simulink model "swingup20112025moi2018a"  (R2018a)
settings: Solver=VariableStepAuto  StartTime=0.0  StopTime=20  RelTol=1e-3
values from neighbouring files (symbols this model uses):
  alphaldotini = 0    [thamsosswingup20112025.m]
  alphalini = 0*pi/180    (= 0)    [thamsosswingup20112025.m]
  bp = 0.005    [calculate_new_K.m]    (also in thamsosswingup20112025.m; verify_quanser_equations.m)
  br = 0.0015    [calculate_new_K.m]    (also in thamsosswingup20112025.m; verify_quanser_equations.m)
  g = 9.81    [calculate_new_K.m]    (also in swingup_control.m = params.g; thamsosswingup20112025.m; verify_quanser_equations.m)
  Jp = mp*(Lp^2)/3    (= 0.000133128)    [calculate_new_K.m]    (also in thamsosswingup20112025.m; verify_quanser_equations.m)
  Jp_cm = params.Jp_cm    [swingup_control.m]    (also in thamsosswingup20112025.m = 3.3282e-05)
  Jr = (mr*r^2)/3    (= 0.000228791666667)    [calculate_new_K.m]    (also in thamsosswingup20112025.m; verify_quanser_equations.m)
  K = (R \ B') * S    [calculate_new_K.m]    (also in lqr_custom.m = R \ (B' * S); swingup_control.m = params.K; thamsosswingup20112025.m = [-3.1623   84.6410   -3.1854    9.2746])
  km = 0.042    [calculate_new_K.m]    (also in thamsosswingup20112025.m)
  Kt = 0.042    [calculate_new_K.m]    (also in thamsosswingup20112025.m)
  l = Lp/2    (= 0.0645)    [calculate_new_K.m]    (also in swingup_control.m = params.l; thamsosswingup20112025.m; verify_quanser_equations.m)
  mp = 0.024    [calculate_new_K.m]    (also in swingup_control.m = params.mp; thamsosswingup20112025.m; verify_quanser_equations.m)
  mr = 0.095    [calculate_new_K.m]    (also in thamsosswingup20112025.m; verify_quanser_equations.m)
  r = 0.085    [calculate_new_K.m]    (also in thamsosswingup20112025.m; verify_quanser_equations.m)
  Rm = 8.4    [calculate_new_K.m]    (also in thamsosswingup20112025.m)
  theta_max = 180*pi/180    (= 3.14159265359)    [thamsosswingup20112025.m]
  thetadotini = 0    [thamsosswingup20112025.m]
  thetaini = 0*pi/180    (= 0)    [thamsosswingup20112025.m]
undefined symbols (not defined in the file or in its folder): Km
libraries: simulink x4, simulink_extras x3
settings Model: Creator=ASUS  LastModifiedBy=ASUS
settings SolverCC: ZeroCrossAlgorithm=Adaptive
settings DataIOCC: ReturnWorkspaceOutputs=on
settings DebuggingCC: IgnoredZcDiagnostic=none  UnconnectedInputMsg=none  UnconnectedOutputMsg=none  UnconnectedLineMsg=none
settings ModelReferenceCC: EnableRefExpFcnMdlSchedulingChecks=off
settings SFSimCC: SimUseLocalCustomCode=on
settings RTWCC: Description=Generic Real-Time Target  RTWUseLocalCustomCode=on

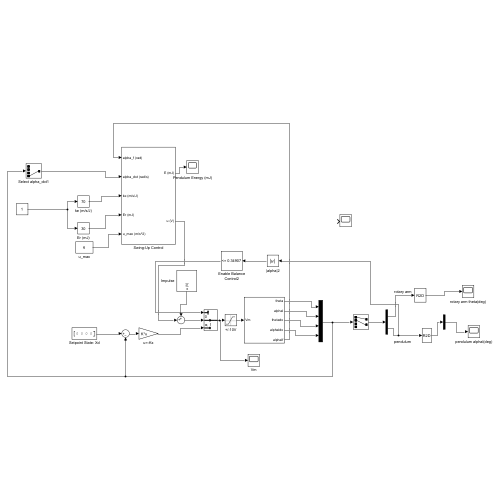
[thumbnail: Simulink's stored preview of the top-level diagram]
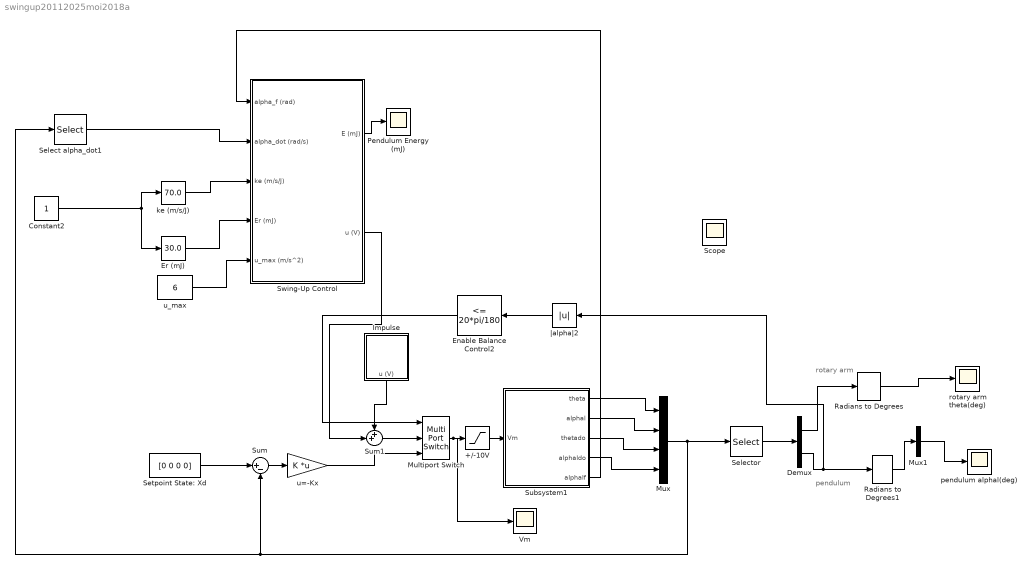
== system swingup20112025moi2018a ==
  note: pendulum
  note: rotary arm
  +/-10V : Saturate  UpperLimit=15  LowerLimit=-15
  Constant2 : Constant
  Demux : Demux  Outputs=2
  Enable Balance Control2 : simulink/Logic and Bit Operations/Compare To Constant  relop=<=  const=20*pi/180  OutDataTypeStr=uint8  ZeroCross=off
  Er (mJ) : simulink/Math Operations/Slider Gain  gain=30.0  low=0  high=100
  Impulse : Subsystem
  Multiport Switch : MultiPortSwitch  DataPortOrder=Zero-based contiguous  Inputs=2  zeroidx=on
  Mux : Mux
  Mux1 : Mux  Inputs=1
  Pendulum Energy (mJ) : Scope
  Radians to Degrees : simulink_extras/Transformations/Radians to Degrees
  Radians to Degrees1 : simulink_extras/Transformations/Radians to Degrees
  Scope : Scope
  Select alpha_dot1 : Selector  InputPortWidth=4  IndexOptions=Index vector (dialog)  Indices=[4]  OutputSizes=1
  Selector : Selector  InputPortWidth=4  IndexOptions=Index vector (dialog)  Indices=[1 2]  OutputSizes=1
  Setpoint State: Xd : Constant  Value=[0 0 0 0]
  Subsystem1 : Subsystem
  Sum : Sum  Inputs=|+-
  Sum1 : Sum  Inputs=++|
  Swing-Up Control : Subsystem
  Vm : Scope
  ke (m/s/J) : simulink/Math Operations/Slider Gain  gain=70.0  low=0  high=100
  pendulum alphal(deg) : Scope
  rotary arm theta(deg) : Scope
  u=-Kx : Gain  Gain=K  Multiplication=Matrix(K*u)
  u_max : Constant  Value=6
  |alpha|2 : Abs
  wires:
  Radians to Degrees1/1 -> Mux1/1
  Demux/1 -> Radians to Degrees/1
  u=-Kx/1 -> Multiport Switch/3
  Selector/1 -> Demux/1
  Enable Balance Control2/1 -> Multiport Switch/1
  Radians to Degrees/1 -> rotary arm theta(deg)/1
  Sum1/1 -> Multiport Switch/2
  Mux1/1 -> pendulum alphal(deg)/1
  Demux/2 -> |alpha|2/1, Radians to Degrees1/1
  Multiport Switch/1 -> Vm/1, +/-10V/1
  Subsystem1/3(thetado) -> Mux/3
  Subsystem1/2(alphal) -> Mux/2
  Subsystem1/1(theta) -> Mux/1
  |alpha|2/1 -> Enable Balance Control2/1
  Mux/1 -> Selector/1, Select alpha_dot1/1, Sum/2
  Subsystem1/4(alphaldo) -> Mux/4
  Swing-Up Control/1(E (mJ)) -> Pendulum Energy (mJ)/1
  Impulse/1(u (V)) -> Sum1/1
  Er (mJ)/1 -> Swing-Up Control/4(Er (mJ))
  ke (m/s/J)/1 -> Swing-Up Control/3(ke (m/s/J))
  Constant2/1 -> Er (mJ)/1, ke (m/s/J)/1
  u_max/1 -> Swing-Up Control/5(u_max (m/s^2))
  Setpoint State: Xd/1 -> Sum/1
  Sum/1 -> u=-Kx/1
  Select alpha_dot1/1 -> Swing-Up Control/2(alpha_dot (rad/s))
  Swing-Up Control/2(u (V)) -> Sum1/2
  +/-10V/1 -> Subsystem1/1(Vm)
  Subsystem1/5(alphalf) -> Swing-Up Control/1(alpha_f (rad))

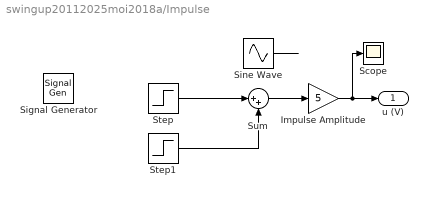
== system swingup20112025moi2018a/Impulse ==
  Impulse Amplitude : Gain  Gain=5
  Scope : Scope
  Signal Generator : SignalGenerator  WaveForm=square  Amplitude=5  Frequency=0.125
  Sine Wave : Sin  Amplitude=6  SampleTime=0
  Step : Step  SampleTime=0
  Step1 : Step  Time=1.1  After=-1  SampleTime=0
  Sum : Sum  Inputs=|++
  u (V) : Outport  VectorParamsAs1DForOutWhenUnconnected=off
  wires:
  Step1/1 -> Sum/2
  Step/1 -> Sum/1
  Sine Wave/1 -> ?
  Impulse Amplitude/1 -> Scope/1, u (V)/1
  Sum/1 -> Impulse Amplitude/1

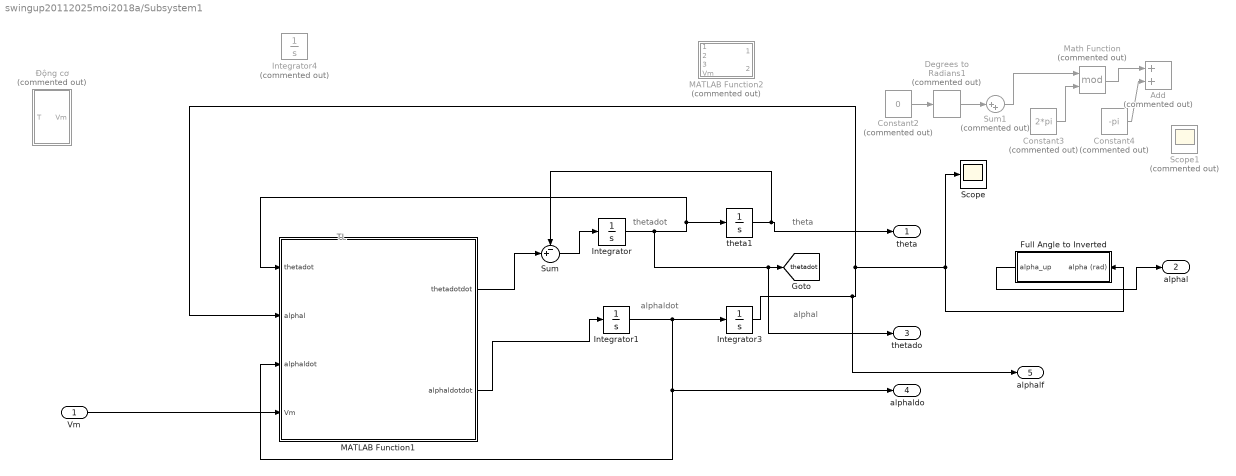
== system swingup20112025moi2018a/Subsystem1 ==
  note: theta
  note: alphaldot
  note: TL
  note: thetadot
  note: alphal
  Vm : Inport
  Add : Sum  Commented=on
  Constant2 : Constant  Commented=on  Value=0
  Constant3 : Constant  Commented=on  Value=2*pi
  Constant4 : Constant  Commented=on  Value=-pi
  Degrees to Radians1 : simulink_extras/Transformations/Degrees to Radians  Commented=on
  Full Angle to Inverted : Subsystem
  Integrator : Integrator  InitialCondition=thetadotini
  Integrator1 : Integrator  InitialCondition=alphaldotini
  Integrator3 : Integrator  InitialCondition=alphalini
  Integrator4 : Integrator  Commented=on  InitialCondition=thetaini
  MATLAB Function1 : MATLAB Function  TreatAsAtomicUnit=on
  MATLAB Function2 : MATLAB Function  Commented=on  TreatAsAtomicUnit=on
  Math Function : Math  Commented=on  Operator=mod  SaturateOnIntegerOverflow=on
  Scope : Scope
  Scope1 : Scope  Commented=on
  Sum : Sum  Inputs=-+|
  Sum1 : Sum  Commented=on  Inputs=|++
  theta1 : Integrator  LimitOutput=on  UpperSaturationLimit=theta_max  LowerSaturationLimit=-theta_max
  Động cơ : Subsystem  Commented=on
  theta : Outport
  alphal : Outport  Port=2
  thetado : Outport  Port=3
  alphaldo : Outport  Port=4
  alphalf : Outport  Port=5
  tag scope: thetadot=global
  wires:
  Integrator/1 -> thetado/1, [thetadot], MATLAB Function1/1(thetadot), theta1/1
  theta1/1 -> Sum/1, theta/1
  Integrator1/1 -> MATLAB Function1/3(alphaldot), alphaldo/1, Integrator3/1
  MATLAB Function1/1(thetadotdot) -> Sum/2
  Constant3/1 -> Math Function/2
  Constant4/1 -> Add/2
  Constant2/1 -> Degrees to Radians1/1
  Math Function/1 -> Add/1
  Sum1/1 -> Math Function/1
  Degrees to Radians1/1 -> Sum1/1
  Sum/1 -> Integrator/1
  Vm/1 -> MATLAB Function1/4(Vm)
  Integrator3/1 -> alphalf/1, Scope/1, Full Angle to Inverted/1(alpha (rad)), MATLAB Function1/2(alphal)
  MATLAB Function1/2(alphaldotdot) -> Integrator1/1
  Full Angle to Inverted/1(alpha_up) -> alphal/1

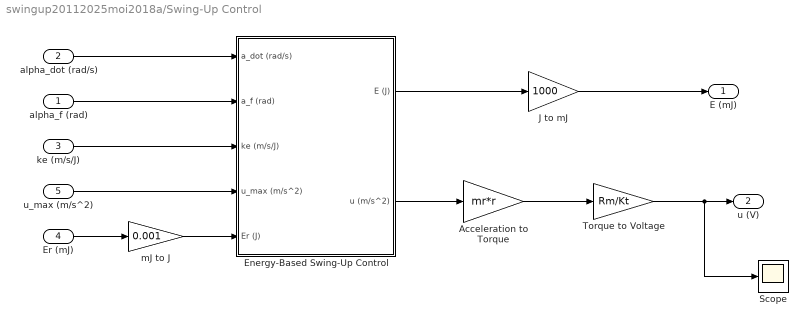
== system swingup20112025moi2018a/Swing-Up Control ==
  alpha_f (rad) : Inport
  alpha_dot (rad/s) : Inport  Port=2
  ke (m/s/J) : Inport  Port=3
  Er (mJ) : Inport  Port=4
  u_max (m/s^2) : Inport  Port=5
  Acceleration to Torque : Gain  Gain=mr*r
  Energy-Based Swing-Up Control : Subsystem
  J to mJ : Gain  Gain=1000
  Scope : Scope
  Torque to Voltage : Gain  Gain=Rm/Kt
  mJ to J : Gain  Gain=0.001
  E (mJ) : Outport  VectorParamsAs1DForOutWhenUnconnected=off
  u (V) : Outport  Port=2  VectorParamsAs1DForOutWhenUnconnected=off
  wires:
  Energy-Based Swing-Up Control/2(u (m/s^2)) -> Acceleration to Torque/1
  Energy-Based Swing-Up Control/1(E (J)) -> J to mJ/1
  alpha_f (rad)/1 -> Energy-Based Swing-Up Control/2(a_f (rad))
  ke (m/s/J)/1 -> Energy-Based Swing-Up Control/3(ke (m/s/J))
  u_max (m/s^2)/1 -> Energy-Based Swing-Up Control/4(u_max (m/s^2))
  Acceleration to Torque/1 -> Torque to Voltage/1
  Er (mJ)/1 -> mJ to J/1
  J to mJ/1 -> E (mJ)/1
  Torque to Voltage/1 -> Scope/1, u (V)/1
  alpha_dot (rad/s)/1 -> Energy-Based Swing-Up Control/1(a_dot (rad/s))
  mJ to J/1 -> Energy-Based Swing-Up Control/5(Er (J))

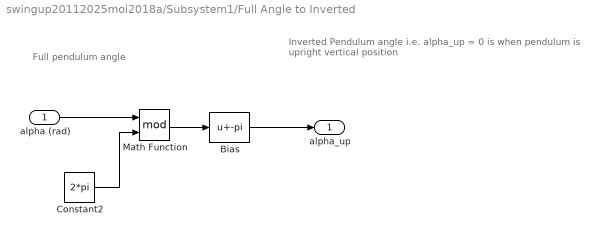
== system swingup20112025moi2018a/Subsystem1/Full Angle to Inverted ==
  note: Inverted Pendulum angle
      | i.e. alpha_up = 0 is when pendulum is upright vertical position
  note: Full pendulum angle
  alpha (rad) : Inport
  Bias : Bias  Bias=-pi
  Constant2 : Constant  Value=2*pi
  Math Function : Math  Operator=mod  SaturateOnIntegerOverflow=on
  alpha_up : Outport  VectorParamsAs1DForOutWhenUnconnected=off
  wires:
  Constant2/1 -> Math Function/2
  alpha (rad)/1 -> Math Function/1
  Bias/1 -> alpha_up/1
  Math Function/1 -> Bias/1

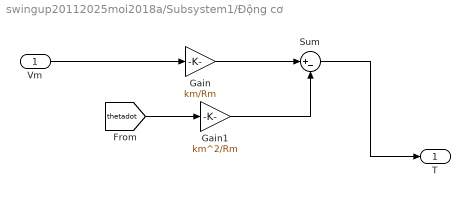
== system swingup20112025moi2018a/Subsystem1/Động cơ ==
  Vm : Inport
  Gain : Gain  Gain=km/Rm
  Gain1 : Gain  Gain=km^2/Rm
  Sum : Sum  Inputs=|+-
  T : Outport
  wires:
  Sum/1 -> T/1
  Gain1/1 -> Sum/2
  Gain/1 -> Sum/1
  Vm/1 -> Gain/1
  [thetadot] -> Gain1/1

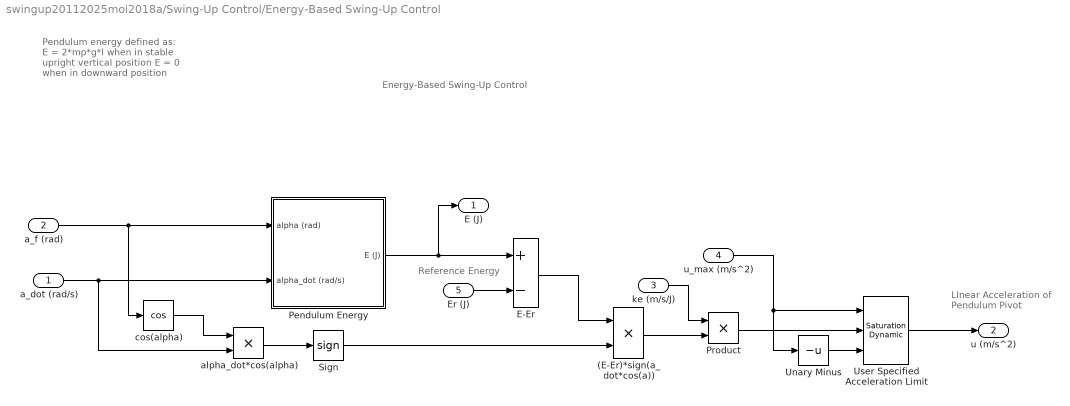
== system swingup20112025moi2018a/Swing-Up Control/Energy-Based Swing-Up Control ==
  note: Energy-Based Swing-Up Control
  note: LInear Acceleration of
      | Pendulum Pivot
  note: Reference Energy
  note: Pendulum energy defined as:
      | E = 2*mp*g*l when in stable upright vertical position
      | E = 0 when in downward position
  a_dot (rad/s) : Inport
  a_f (rad) : Inport  Port=2
  ke (m/s/J) : Inport  Port=3
  u_max (m/s^2) : Inport  Port=4
  Er (J) : Inport  Port=5
  (E-Er)*sign(a_dot*cos(a)) : Product  RndMeth=Zero
  E-Er : Sum  Inputs=+-
  Pendulum Energy : Subsystem
  Product : Product  RndMeth=Zero
  Sign : Signum
  Unary Minus : UnaryMinus
  User Specified Acceleration Limit : simulink/Discontinuities/Saturation Dynamic  OutMin=[]  OutMax=[]  OutDataTypeStr=Inherit: Same as second input  OutDataType=fixdt(1, 16)  OutScaling=2^-10  DoSatur=off
  alpha_dot*cos(alpha) : Product  RndMeth=Zero
  cos(alpha) : Trigonometry  Operator=cos
  E (J) : Outport  VectorParamsAs1DForOutWhenUnconnected=off
  u (m/s^2) : Outport  Port=2  VectorParamsAs1DForOutWhenUnconnected=off
  wires:
  a_f (rad)/1 -> Pendulum Energy/1(alpha (rad)), cos(alpha)/1
  Sign/1 -> (E-Er)*sign(a_dot*cos(a))/2
  alpha_dot*cos(alpha)/1 -> Sign/1
  cos(alpha)/1 -> alpha_dot*cos(alpha)/1
  E-Er/1 -> (E-Er)*sign(a_dot*cos(a))/1
  Pendulum Energy/1(E (J)) -> E (J)/1, E-Er/1
  a_dot (rad/s)/1 -> alpha_dot*cos(alpha)/2, Pendulum Energy/2(alpha_dot (rad/s))
  (E-Er)*sign(a_dot*cos(a))/1 -> Product/2
  Er (J)/1 -> E-Er/2
  ke (m/s/J)/1 -> Product/1
  Product/1 -> User Specified Acceleration Limit/2
  u_max (m/s^2)/1 -> User Specified Acceleration Limit/1, Unary Minus/1
  Unary Minus/1 -> User Specified Acceleration Limit/3
  User Specified Acceleration Limit/1 -> u (m/s^2)/1

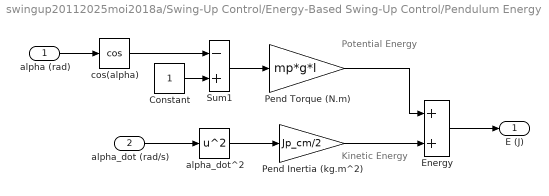
== system swingup20112025moi2018a/Swing-Up Control/Energy-Based Swing-Up Control/Pendulum Energy ==
  note: Kinetic Energy
  note: Potential Energy
  alpha (rad) : Inport
  alpha_dot (rad/s) : Inport  Port=2
  Constant : Constant
  Energy : Sum  SaturateOnIntegerOverflow=on
  Pend Inertia (kg.m^2) : Gain  Gain=Jp_cm/2
  Pend Torque (N.m) : Gain  Gain=mp*g*l
  Sum1 : Sum  Inputs=-+  SaturateOnIntegerOverflow=on
  alpha_dot^2 : Math  Operator=square  SaturateOnIntegerOverflow=on
  cos(alpha) : Trigonometry  Operator=cos
  E (J) : Outport  VectorParamsAs1DForOutWhenUnconnected=off
  wires:
  Sum1/1 -> Pend Torque (N.m)/1
  Constant/1 -> Sum1/2
  Pend Inertia (kg.m^2)/1 -> Energy/2
  alpha_dot^2/1 -> Pend Inertia (kg.m^2)/1
  Pend Torque (N.m)/1 -> Energy/1
  alpha (rad)/1 -> cos(alpha)/1
  alpha_dot (rad/s)/1 -> alpha_dot^2/1
  Energy/1 -> E (J)/1
  cos(alpha)/1 -> Sum1/1

== matlab function swingup20112025moi2018a/Subsystem1/MATLAB Function1 ==
  data: thetadotdot output; alphaldotdot output; thetadot input; alphal input; alphaldot input; Vm input; Jr parameter; br parameter; bp parameter; g parameter; l parameter; mp parameter; r parameter; Jp parameter; Kt parameter; Rm parameter; km parameter
function [thetadotdot,alphaldotdot] = fcn(thetadot,alphal, alphaldot,Vm,Jr, br, bp, g, l, mp, r, Jp,Kt, Rm, km)
 
thetadotdot = (Jp*(Kt/Rm)*(Vm-km*thetadot) - Jp*br*thetadot - 2*Jp^2*alphaldot*thetadot*cos(alphal)*sin(alphal) + alphaldot*bp*l*mp*r*cos(alphal) + g*l^2*mp^2*r*cos(alphal)*sin(alphal) + Jp*alphaldot^2*l*mp*r*sin(alphal) - Jp*l*mp*r*thetadot^2*cos(alphal)^2*sin(alphal))/(Jp^2*sin(alphal)^2 + Jr*Jp - l^2*mp^2*r^2*cos(alphal)^2);
 
alphaldotdot = -(Jr*alphaldot*bp + Jp*alphaldot*bp*sin(alphal)^2 - Jp^2*thetadot^2*cos(alphal)*sin(alphal)^3 + Jp*g*l*mp*sin(alphal)^3 - Jp*Jr*thetadot^2*cos(alphal)*sin(alphal) + Jr*g*l*mp*sin(alphal) + (Kt/Rm)*(Vm-km*thetadot)*l*mp*r*cos(alphal) + alphaldot^2*l^2*mp^2*r^2*cos(alphal)*sin(alphal) - br*l*mp*r*thetadot*cos(alphal) - 2*Jp*alphaldot*l*mp*r*thetadot*cos(alphal)^2*sin(alphal))/(Jp^2*sin(alphal)^2 + Jr*Jp - l^2*mp^2*r^2*cos(alphal)^2);

== matlab function swingup20112025moi2018a/Subsystem1/MATLAB Function2 ==
  data: thetadotdot output; alphaldotdot output; thetadot input; alphal input; alphaldot input; Vm input; Jr parameter; br parameter; bp parameter; g parameter; l parameter; mp parameter; r parameter; Jp parameter; Kt parameter; Rm parameter; Km parameter
function [thetadotdot,alphaldotdot] = fcn(thetadot,alphal, alphaldot,Vm,Jr, br, bp, g, l, mp, r, Jp,Kt, Rm, Km)
 
 
 
thetadotdot = (2*Jp*Kt*Vm + 2*Kt*l^2*mp*Vm - 2*Jp*Km*Kt*thetadot - 2*Jp*Rm*br*thetadot - 2*Km*Kt*l^2*mp*thetadot - 2*Rm*br*l^2*mp*thetadot + 2*Rm*alphaldot^2*l^3*mp^2*r*sin(alphal) - 2*Rm*alphaldot*l^4*mp^2*thetadot*sin(2*alphal) + Rm*g*l^2*mp^2*r*sin(2*alphal) - 2*Jp*Rm*alphaldot*l^2*mp*thetadot*sin(2*alphal) + 2*Rm*alphaldot*bp*l*mp*r*cos(alphal) + 2*Jp*Rm*alphaldot^2*l*mp*r*sin(alphal) + 2*Rm*l^3*mp^2*r*thetadot^2*sin(alphal)*(sin(alphal)^2 - 1))/(2*Rm*(l^4*mp^2*sin(alphal)^2 + l^2*mp^2*r^2*sin(alphal)^2 + Jp*l^2*mp*sin(alphal)^2 + Jr*l^2*mp + Jp*mp*r^2 + Jp*Jr));
 
 
alphaldotdot = -(2*Jr*Rm*alphaldot*bp + 2*Rm*alphaldot*bp*mp*r^2 + 2*Rm*g*l^3*mp^2*sin(alphal)^3 + Rm*alphaldot^2*l^2*mp^2*r^2*sin(2*alphal) + 2*Jr*Rm*g*l*mp*sin(alphal) - 2*Rm*l^4*mp^2*thetadot^2*cos(alphal)*sin(alphal)^3 - Rm*l^2*mp^2*r^2*thetadot^2*sin(2*alphal) + 2*Kt*l*mp*r*Vm*cos(alphal) - Jr*Rm*l^2*mp*thetadot^2*sin(2*alphal) + 2*Rm*alphaldot*bp*l^2*mp*sin(alphal)^2 + 2*Rm*g*l*mp^2*r^2*sin(alphal) - 2*Km*Kt*l*mp*r*thetadot*cos(alphal) - 2*Rm*br*l*mp*r*thetadot*cos(alphal) + 4*Rm*alphaldot*l^3*mp^2*r*thetadot*sin(alphal)*(sin(alphal)^2 - 1))/(2*Rm*(l^4*mp^2*sin(alphal)^2 + l^2*mp^2*r^2*sin(alphal)^2 + Jp*l^2*mp*sin(alphal)^2 + Jr*l^2*mp + Jp*mp*r^2 + Jp*Jr));
